simulink library "vmc"  (R2021b)
settings: Solver=VariableStepAuto  StartTime=0.0  StopTime=10.0  RelTol=1e-3
undefined symbols (not defined in the file or in its folder): AVMC_ACCDeltaTqIGain_X_kph, AVMC_ACCDeltaTqIGain_Y_mps2, AVMC_ACCDeltaTqPGain_X_kph, AVMC_ACCDeltaTqPGain_Y_kph, AVMC_ACCLongSteadyCtrl_X_kph, AVMC_AggressJerkPCT4AT_X_kph, AVMC_AggressJerkPCT_X_kph, AVMC_AggressLimitPCT4AT_X_kph, AVMC_AggressLimitPCT_X_kph, AVMC_CCLongSteadyCtrl_X_kph, AVMC_DISCDeltaTqIGain_X_kph, AVMC_DISCDeltaTqIGain_Y_mps2, AVMC_DISCDeltaTqPGain_X_kph, AVMC_DISCDeltaTqPGain_Y_kph, AVMC_DISCTrunAccJerk_X_s, AVMC_DISCTrunAccLimit_X_s, AVMC_ESCRegenOut_X_kph, AVMC_ESCRegenOut_Y_Deg, AVMC_ESCRegenOutEnSpd_X_Deg, AVMC_ISOAccLimit_X_mps, AVMC_ISODecLimit_X_mps, AVMC_ISOJerk_X_mps, AVMC_LatESCRegenOut_X_kph, AVMC_LatESCRegenOut_Y_Deg, AVMC_LongAccDeadZone_X_kph, AVMC_LongAccFiltTsforP2_X_Gps, AVMC_MCPresBaseTq_X_bar, AVMC_MSALongSteadyCtrl_X_kph, AVMC_MSAPedalOvrd2_X_kph, AVMC_MSAPedalOvrd_X_kph, AVMC_MSASpdBand_X_kph, AVMC_MSATqDownEndTq_X_kph, AVMC_MSATqDownTime_X_kph, AVMC_OPDDisSlideRate_X_Deg, AVMC_RDCDetectTime_X_kph, AVMC_RDCDetectTime_Y_pct, AVMC_RDCEnSlideRate_X_Deg, AVMC_RearWhlTqRatio_X_Nm, AVMC_RearWhlTqRatio_Y_gps, AVMC_RearWhlTqSlipGain_X_rat, AVMC_RearWhlTqSlipGain_Y_kph, AVMC_RearWhlTqSTRGGain_X_deg, AVMC_RearWhlTqSTRGGain_Y_kph, AVMC_RWSRrTSA2RWSPos_X_deg, AVMC_RWSSAS2FrtTSA_X_deg, AVMC_RWSVehSPD2RWSCoef_X_kph, AVMC_SoftJerkPCT_X_kph, AVMC_SoftLimitPCT_X_kph, AVMC_StESCYaw_X_kph, AVMC_StESCYaw_Y_Deg, AVMC_StESCYawCom_X_kph, AVMC_StESCYawCom_Y_Gps, AVMC_TMSpdBaseTq_X_rpm, AVMC_VehHoldBDecMap_X_kph, AVMC_VehHoldDecCtrlTime_X_kph, AVMC_VehHoldMCPPass_X_deg, C_TASK_10MS_S, C_TASK_5MS_S, DEG2RAD, ENUM_ACCAVAIL_AVAILABLE ... (+409)
libraries: hcu_lib x74, simulink x68, simulink_extras x3, $bdroot x2
(part 11 of 15)

== system vmc/VMC/VMC/SafetyControl/SafetyControlJudgement ==
  VINP_VehSpeed_kph : Inport
  VVMC_LFWhlSpeedRollAve_kph : Inport  Port=2
  VVMC_RFWhlSpeedRollAve_kph : Inport  Port=3
  VVMC_LRWhlSpeedRollAve_kph : Inport  Port=4
  VVMC_RRWhlSpeedRollAve_kph : Inport  Port=5
  VINP_LFRawWhlSpeedV_flg : Inport  Port=6
  VINP_RFRawWhlSpeedV_flg : Inport  Port=7
  VINP_LRRawWhlSpeedV_flg : Inport  Port=8
  VINP_RRRawWhlSpeedV_flg : Inport  Port=9
  VVMC_LatAccRollAve_Gps : Inport  Port=10
  VINP_LatAccelV_flg : Inport  Port=11
  VVMC_FeatArbitrFinal_enum : Inport  Port=12
  Cast To Single{,1..3} (4 alike) : DataTypeConversion  OutDataTypeStr=boolean
  Constant18 : Constant  Value=C_TASK_10MS_S
  Constant20 : Constant  Value=KVMC_SafetyCtrlAllowTime_s
  Constant21 : Constant  Value=TRUE
  Constant22 : Constant  Value=FALSE
  FrontRearSlipRatio : Subsystem
  LateralAccelerationControl : Subsystem
  NOT : Logic  Operator=NOT  AllPortsSameDT=off  OutDataTypeStr=boolean
  RearWheelSlipRatio : Subsystem
  Relational Operator16 : RelationalOperator  OutDataTypeStr=boolean  RndMeth=Simplest
  SafetyControlJudgement : Subsystem
  SingleWheelSlipRatio : Subsystem
  Timer : hcu_lib/Basic_Blocks/Timer
  u2 > 0 (1) : Switch  Criteria=u2 > Threshold
  VVMC_SafetyCtrl_flg : Outport
  VVMC_FrontRearSlipRatioCtrl_flg : Outport  Port=2
  VVMC_RearWhlSlipRatioCtrl_flg : Outport  Port=3
  VVMC_SingleWhlSlipRatioCtrl_flg : Outport  Port=4
  VVMC_LatAccCtrl_flg : Outport  Port=5
  wires:
  [VVMC_FeatArbitrFinal_enum] -> SafetyControlJudgement/5(VVMC_FeatArbitrFinal_enum)
  VVMC_FeatArbitrFinal_enum/1 -> [VVMC_FeatArbitrFinal_enum]
  Constant18/1 -> Timer/3
  Constant22/1 -> u2 > 0 (1)/3
  Relational Operator16/1 -> u2 > 0 (1)/2
  Timer/1 -> Relational Operator16/1
  Constant20/1 -> Relational Operator16/2, Timer/4
  Constant21/1 -> u2 > 0 (1)/1
  SafetyControlJudgement/1("VVMC_SafetyCtrl_flg ") -> NOT/1, Timer/1
  NOT/1 -> Timer/2
  u2 > 0 (1)/1 -> [VVMC_SafetyCtrl_flg]
  [VVMC_LatAccCtrl_flg] -> VVMC_LatAccCtrl_flg/1
  [VVMC_SingleWhlSlipRatioCtrl_flg] -> VVMC_SingleWhlSlipRatioCtrl_flg/1
  [VVMC_RearWhlSlipRatioCtrl_flg] -> VVMC_RearWhlSlipRatioCtrl_flg/1
  [VVMC_FrontRearSlipRatioCtrl_flg] -> VVMC_FrontRearSlipRatioCtrl_flg/1
  [VVMC_LatAccCtrl_flg] -> SafetyControlJudgement/4(VVMC_LatAccCtrl_flg)
  Cast To Single3/1 -> [VVMC_LatAccCtrl_flg]  "VVMC_LatAccCtrl_flg"
  LateralAccelerationControl/1(VVMC_LatAccCtrl_flg) -> Cast To Single3/1
  [VINP_LatAccelV_flg] -> LateralAccelerationControl/2(VINP_LatAccelV_flg)
  [VVMC_LatAccRollAve_Gps] -> LateralAccelerationControl/1(VVMC_LatAccRollAve_Gps)
  VVMC_LatAccRollAve_Gps/1 -> [VVMC_LatAccRollAve_Gps]
  VINP_LatAccelV_flg/1 -> [VINP_LatAccelV_flg]
  Cast To Single2/1 -> [VVMC_SingleWhlSlipRatioCtrl_flg]  "VVMC_SingleWhlSlipRatioCtrl_flg"
  Cast To Single1/1 -> [VVMC_RearWhlSlipRatioCtrl_flg]  "VVMC_RearWhlSlipRatioCtrl_flg"
  Cast To Single/1 -> [VVMC_FrontRearSlipRatioCtrl_flg]  "VVMC_FrontRearSlipRatioCtrl_flg"
  [VVMC_SafetyCtrl_flg] -> VVMC_SafetyCtrl_flg/1
  [VVMC_SingleWhlSlipRatioCtrl_flg] -> SafetyControlJudgement/3(VVMC_SingleWhlSlipRatioCtrl_flg)
  [VVMC_RearWhlSlipRatioCtrl_flg] -> SafetyControlJudgement/2(VVMC_RearWhlSlipRatioCtrl_flg)
  [VVMC_FrontRearSlipRatioCtrl_flg] -> SafetyControlJudgement/1(VVMC_FrontRearSlipRatioCtrl_flg)
  [VINP_VehSpeed_kph] -> SingleWheelSlipRatio/1(VINP_VehSpeed_kph)
  [VVMC_LFWhlSpeedRollAve_kph] -> SingleWheelSlipRatio/2(VVMC_LFWhlSpeedRollAve_kph)
  [VVMC_RFWhlSpeedRollAve_kph] -> SingleWheelSlipRatio/3(VVMC_RFWhlSpeedRollAve_kph)
  [VVMC_LRWhlSpeedRollAve_kph] -> SingleWheelSlipRatio/4(VVMC_LRWhlSpeedRollAve_kph)
  [VVMC_RRWhlSpeedRollAve_kph] -> SingleWheelSlipRatio/5(VVMC_RRWhlSpeedRollAve_kph)
  [VINP_LFRawWhlSpeedV_flg] -> SingleWheelSlipRatio/6(VINP_LFRawWhlSpeedV_flg)
  [VINP_RFRawWhlSpeedV_flg] -> SingleWheelSlipRatio/7(VINP_RFRawWhlSpeedV_flg)
  [VINP_LRRawWhlSpeedV_flg] -> SingleWheelSlipRatio/8(VINP_LRRawWhlSpeedV_flg)
  [VINP_RRRawWhlSpeedV_flg] -> SingleWheelSlipRatio/9(VINP_RRRawWhlSpeedV_flg)
  SingleWheelSlipRatio/1(VVMC_SingleWhlSlipRatioCtrl_flg) -> Cast To Single2/1
  [VVMC_LRWhlSpeedRollAve_kph] -> RearWheelSlipRatio/1(VVMC_LRWhlSpeedRollAve_kph)
  [VVMC_RRWhlSpeedRollAve_kph] -> RearWheelSlipRatio/2(VVMC_RRWhlSpeedRollAve_kph)
  [VINP_LRRawWhlSpeedV_flg] -> RearWheelSlipRatio/3(VINP_LRRawWhlSpeedV_flg)
  [VINP_RRRawWhlSpeedV_flg] -> RearWheelSlipRatio/4(VINP_RRRawWhlSpeedV_flg)
  RearWheelSlipRatio/1("VVMC_RearWhlSlipRatioCtrl_flg ") -> Cast To Single1/1
  FrontRearSlipRatio/1("VVMC_FrontRearSlipRatioCtrl_flg ") -> Cast To Single/1
  [VINP_RRRawWhlSpeedV_flg] -> FrontRearSlipRatio/8(VINP_RRRawWhlSpeedV_flg)
  [VINP_LRRawWhlSpeedV_flg] -> FrontRearSlipRatio/7(VINP_LRRawWhlSpeedV_flg)
  [VINP_RFRawWhlSpeedV_flg] -> FrontRearSlipRatio/6(VINP_RFRawWhlSpeedV_flg)
  [VINP_LFRawWhlSpeedV_flg] -> FrontRearSlipRatio/5(VINP_LFRawWhlSpeedV_flg)
  [VVMC_RRWhlSpeedRollAve_kph] -> FrontRearSlipRatio/4(VVMC_RRWhlSpeedRollAve_kph)
  [VVMC_LRWhlSpeedRollAve_kph] -> FrontRearSlipRatio/3(VVMC_LRWhlSpeedRollAve_kph)
  [VVMC_RFWhlSpeedRollAve_kph] -> FrontRearSlipRatio/2(VVMC_RFWhlSpeedRollAve_kph)
  [VVMC_LFWhlSpeedRollAve_kph] -> FrontRearSlipRatio/1(VVMC_LFWhlSpeedRollAve_kph)
  VINP_RRRawWhlSpeedV_flg/1 -> [VINP_RRRawWhlSpeedV_flg]
  VINP_LRRawWhlSpeedV_flg/1 -> [VINP_LRRawWhlSpeedV_flg]
  VINP_RFRawWhlSpeedV_flg/1 -> [VINP_RFRawWhlSpeedV_flg]
  VINP_LFRawWhlSpeedV_flg/1 -> [VINP_LFRawWhlSpeedV_flg]
  VVMC_LFWhlSpeedRollAve_kph/1 -> [VVMC_LFWhlSpeedRollAve_kph]
  VVMC_RFWhlSpeedRollAve_kph/1 -> [VVMC_RFWhlSpeedRollAve_kph]
  VVMC_LRWhlSpeedRollAve_kph/1 -> [VVMC_LRWhlSpeedRollAve_kph]
  VVMC_RRWhlSpeedRollAve_kph/1 -> [VVMC_RRWhlSpeedRollAve_kph]
  VINP_VehSpeed_kph/1 -> [VINP_VehSpeed_kph]

== system vmc/VMC/VMC/SafetyControl/VehSpdRollingAverage ==
  VINP_VehSpeed_kph : Inport
  Constant3 : Constant  Value=ONE_INT
  Constant4 : Constant  Value=KVMC_VehSpdRollAveLevel_enum
  Constant5 : Constant  Value=ZERO_FLOAT
  RollingAverage : Stateflow chart  TreatAsAtomicUnit=on
  VVMC_VehSpdRollAve_kph : Outport
  wires:
  [VVMC_VehSpdRollAve_kph] -> VVMC_VehSpdRollAve_kph/1
  VINP_VehSpeed_kph/1 -> [VINP_VehSpeed_kph]  "VINP_VehSpeed_kph"
  RollingAverage/1(VVMC_VehSpdRollAve_kph) -> [VVMC_VehSpdRollAve_kph]  "VVMC_VehSpdRollAve_kph"
  [VINP_VehSpeed_kph] -> RollingAverage/4(VINP_VehSpeed_kph)
  Constant3/1 -> RollingAverage/3(ONE_INT)
  Constant5/1 -> RollingAverage/2(ZERO_FLOAT)
  Constant4/1 -> RollingAverage/1(KVMC_VehSpdRollAveLevel_enum)

== system vmc/VMC/VMC/SafetyControl/WheelSpeedRollingAverage ==
  VINP_LFRawWhlSpeed_kph : Inport
  VINP_RFRawWhlSpeed_kph : Inport  Port=2
  VINP_LRRawWhlSpeed_kph : Inport  Port=3
  VINP_RRRawWhlSpeed_kph : Inport  Port=4
  Constant{3,7,12,16} (4 alike) : Constant  Value=ONE_INT
  Constant{4,8,13,17} (4 alike) : Constant  Value=KVMC_WhlSpdRollAveLevel_enum
  Constant{5,9,14,18} (4 alike) : Constant  Value=ZERO_FLOAT
  RollingAverage : Stateflow chart  TreatAsAtomicUnit=on
  RollingAverage1 : Stateflow chart  TreatAsAtomicUnit=on
  RollingAverage2 : Stateflow chart  TreatAsAtomicUnit=on
  RollingAverage3 : Stateflow chart  TreatAsAtomicUnit=on
  VVMC_LFWhlSpeedRollAve_kph : Outport
  VVMC_RFWhlSpeedRollAve_kph : Outport  Port=2
  VVMC_LRWhlSpeedRollAve_kph : Outport  Port=3
  VVMC_RRWhlSpeedRollAve_kph : Outport  Port=4
  wires:
  [VVMC_RRWhlSpeedRollAve_kph] -> VVMC_RRWhlSpeedRollAve_kph/1
  [VVMC_LRWhlSpeedRollAve_kph] -> VVMC_LRWhlSpeedRollAve_kph/1
  [VVMC_RFWhlSpeedRollAve_kph] -> VVMC_RFWhlSpeedRollAve_kph/1
  [VVMC_LFWhlSpeedRollAve_kph] -> VVMC_LFWhlSpeedRollAve_kph/1
  VINP_RFRawWhlSpeed_kph/1 -> [VINP_RFRawWhlSpeed_kph]
  VINP_LFRawWhlSpeed_kph/1 -> [VINP_LFRawWhlSpeed_kph]
  VINP_RRRawWhlSpeed_kph/1 -> [VINP_RRRawWhlSpeed_kph]
  VINP_LRRawWhlSpeed_kph/1 -> [VINP_LRRawWhlSpeed_kph]
  Constant4/1 -> RollingAverage/1(KVMC_WhlSpdRollAveLevel_enum)
  Constant5/1 -> RollingAverage/2(ZERO_FLOAT)
  Constant3/1 -> RollingAverage/3(ONE_INT)
  [VINP_LFRawWhlSpeed_kph] -> RollingAverage/4(VINP_LFRawWhlSpeed_kph)
  RollingAverage/1(VVMC_LFWhlSpeedRollAve_kph) -> [VVMC_LFWhlSpeedRollAve_kph]
  [VINP_RFRawWhlSpeed_kph] -> RollingAverage1/4(VINP_RFRawWhlSpeed_kph)
  Constant7/1 -> RollingAverage1/3(ONE_INT)
  Constant9/1 -> RollingAverage1/2(ZERO_FLOAT)
  Constant8/1 -> RollingAverage1/1(KVMC_WhlSpdRollAveLevel_enum)
  Constant17/1 -> RollingAverage3/1(KVMC_WhlSpdRollAveLevel_enum)
  Constant18/1 -> RollingAverage3/2(ZERO_FLOAT)
  Constant16/1 -> RollingAverage3/3(ONE_INT)
  [VINP_RRRawWhlSpeed_kph] -> RollingAverage3/4(VINP_RRRawWhlSpeed_kph)
  RollingAverage2/1(VVMC_LRWhlSpeedRollAve_kph) -> [VVMC_LRWhlSpeedRollAve_kph]
  [VINP_LRRawWhlSpeed_kph] -> RollingAverage2/4(VINP_LRRawWhlSpeed_kph)
  Constant12/1 -> RollingAverage2/3(ONE_INT)
  Constant14/1 -> RollingAverage2/2(ZERO_FLOAT)
  Constant13/1 -> RollingAverage2/1(KVMC_WhlSpdRollAveLevel_enum)
  RollingAverage1/1(VVMC_RFWhlSpeedRollAve_kph) -> [VVMC_RFWhlSpeedRollAve_kph]
  RollingAverage3/1(VVMC_RRWhlSpeedRollAve_kph) -> [VVMC_RRWhlSpeedRollAve_kph]

== system vmc/VMC/VMC/Slide Rate  Calculation/4Wheel Calculation ==
  VINP_LFRawWhlSpeed_kph : Inport
  VINP_RFRawWhlSpeed_kph : Inport  Port=2
  VINP_LRRawWhlSpeed_kph : Inport  Port=3
  VINP_RRRawWhlSpeed_kph : Inport  Port=4
  VVMC_LongAcc_Gps : Inport  Port=5
  task_time_s : Inport  Port=6
  VINP_VehSpeed_kph : Inport  Port=7
  VTQD_AfterAvailableTqDemFr_Nm : Inport  Port=8
  VTQD_AfterAvailableTqDemRr_Nm : Inport  Port=9
  VTQD_GearActualPosn_enum : Inport  Port=10
  VINP_LongAccel_Gps : Inport  Port=11
  Constant3 : Constant  Value=KVMC_4WheelLongAccSW_flg
  Determination : Subsystem
  LF Wheel : Subsystem
  LR Wheel : Subsystem
  RF Wheel : Subsystem
  RR Wheel : Subsystem
  Switch : Switch  Criteria=u2 > Threshold
  VVMC_LF4WhlSpdSlideRate_pct : Outport
  VVMC_RF4WhlSpdSlideRate_pct : Outport  Port=2
  VVMC_LR4WhlSpdSlideRate_pct : Outport  Port=3
  VVMC_RR4WhlSpdSlideRate_pct : Outport  Port=4
  VVMC_PredictVehSpd_kph : Outport  Port=5
  VVMC_4WhlSpdSlideRate_pct : Outport  Port=6
  VVMC_AllWhlSkid_flg : Outport  Port=7
  wires:
  [VVMC_4WhlSpdSlideRate_pct] -> VVMC_4WhlSpdSlideRate_pct/1
  [VVMC_PredictVehSpd_kph] -> VVMC_PredictVehSpd_kph/1
  VINP_VehSpeed_kph/1 -> [VINP_VehSpeed_kph]
  task_time_s/1 -> [task_time_s]
  [VVMC_LR4WhlSpdSlideRate_pct] -> VVMC_LR4WhlSpdSlideRate_pct/1
  [VVMC_RR4WhlSpdSlideRate_pct] -> VVMC_RR4WhlSpdSlideRate_pct/1
  [VVMC_RF4WhlSpdSlideRate_pct] -> VVMC_RF4WhlSpdSlideRate_pct/1
  [VVMC_LF4WhlSpdSlideRate_pct] -> VVMC_LF4WhlSpdSlideRate_pct/1
  VINP_LRRawWhlSpeed_kph/1 -> [VINP_LRRawWhlSpeed_kph]
  VINP_LFRawWhlSpeed_kph/1 -> [VINP_LFRawWhlSpeed_kph]
  VINP_RFRawWhlSpeed_kph/1 -> [VINP_RFRawWhlSpeed_kph]
  VINP_RRRawWhlSpeed_kph/1 -> [VINP_RRRawWhlSpeed_kph]
  [VVMC_AllWhlSkid_flg] -> VVMC_AllWhlSkid_flg/1
  VTQD_AfterAvailableTqDemFr_Nm/1 -> [VTQD_AfterAvailableTqDemFr_Nm]
  VTQD_AfterAvailableTqDemRr_Nm/1 -> [VTQD_AfterAvailableTqDemRr_Nm]
  VTQD_GearActualPosn_enum/1 -> [VTQD_GearActualPosn_enum]
  [VVMC_LRPreVehSpd_kph] -> Determination/17(VVMC_LRPreVehSpd_kph)
  [VVMC_4WheelLongAcc_Gps] -> LF Wheel/1(VVMC_4WheelLongAcc_Gps)
  [VINP_RRRawWhlSpeed_kph] -> RR Wheel/3(VINP_RRRawWhlSpeed_kph)
  [VINP_LRRawWhlSpeed_kph] -> LR Wheel/3(VINP_LRRawWhlSpeed_kph)
  [VINP_RFRawWhlSpeed_kph] -> RF Wheel/3(VINP_RFRawWhlSpeed_kph)
  [VTQD_GearActualPosn_enum] -> RF Wheel/4(VTQD_GearActualPosn_enum)
  LF Wheel/1(VVMC_LFPreVehSpd_kph) -> [VVMC_LFPreVehSpd_kph]
  RR Wheel/1(VVMC_RRPreVehSpd_kph) -> [VVMC_RRPreVehSpd_kph]
  [VTQD_GearActualPosn_enum] -> LR Wheel/4(VTQD_GearActualPosn_enum)
  [VVMC_LF4WhlSpdSlideRate_pct] -> Determination/9(VVMC_LF4WhlSpdSlideRate_pct)
  [VVMC_RRWhlSkid_flg] -> Determination/8(VVMC_RRWhlSkid_flg)
  [VINP_LFRawWhlSpeed_kph] -> LF Wheel/3(VINP_LFRawWhlSpeed_kph)
  [task_time_s] -> RR Wheel/2(task_time_s)
  [task_time_s] -> RF Wheel/2(task_time_s)
  [VVMC_RR4WhlSpdSlideRate_pct] -> Determination/12(VVMC_RR4WhlSpdSlideRate_pct)
  RR Wheel/3(VVMC_RR4WhlSpdSlideRate_pct) -> [VVMC_RR4WhlSpdSlideRate_pct]
  [VTQD_AfterAvailableTqDemFr_Nm] -> Determination/13(VTQD_AfterAvailableTqDemFr_Nm)
  [VVMC_LR4WhlSpdSlideRate_pct] -> Determination/11(VVMC_LR4WhlSpdSlideRate_pct)
  [VTQD_GearActualPosn_enum] -> Determination/4(VTQD_GearActualPosn_enum)
  [task_time_s] -> Determination/2(task_time_s)
  [VVMC_LFWhlSkid_flg] -> Determination/5(VVMC_LFWhlSkid_flg)
  [VINP_VehSpeed_kph] -> Determination/3(VINP_VehSpeed_kph)
  [VVMC_RRPreVehSpd_kph] -> Determination/18(VVMC_RRPreVehSpd_kph)
  Determination/2(VVMC_AllWhlSkid_flg) -> [VVMC_AllWhlSkid_flg]
  Determination/1(VVMC_PredictVehSpd_kph) -> [VVMC_PredictVehSpd_kph]
  Determination/3(VVMC_4WhlSpdSlideRate_pct) -> [VVMC_4WhlSpdSlideRate_pct]
  [VVMC_RFWhlSkid_flg] -> Determination/6(VVMC_RFWhlSkid_flg)
  LR Wheel/3(VVMC_LR4WhlSpdSlideRate_pct) -> [VVMC_LR4WhlSpdSlideRate_pct]
  LR Wheel/2(VVMC_LRWhlSkid_flg) -> [VVMC_LRWhlSkid_flg]
  [VVMC_LRWhlSkid_flg] -> Determination/7(VVMC_LRWhlSkid_flg)
  RF Wheel/1(VVMC_RFPreVehSpd_kph) -> [VVMC_RFPreVehSpd_kph]
  [task_time_s] -> LR Wheel/2(task_time_s)
  [VVMC_RFPreVehSpd_kph] -> Determination/16(VVMC_RFPreVehSpd_kph)
  LR Wheel/1(VVMC_LRPreVehSpd_kph) -> [VVMC_LRPreVehSpd_kph]
  [VVMC_4WheelLongAcc_Gps] -> RF Wheel/1(VVMC_4WheelLongAcc_Gps)
  RR Wheel/2(VVMC_RRWhlSkid_flg) -> [VVMC_RRWhlSkid_flg]
  [VVMC_LFPreVehSpd_kph] -> Determination/15(VVMC_LFPreVehSpd_kph)
  [VVMC_RF4WhlSpdSlideRate_pct] -> Determination/10(VVMC_RF4WhlSpdSlideRate_pct)
  [VTQD_AfterAvailableTqDemRr_Nm] -> Determination/14(VTQD_AfterAvailableTqDemRr_Nm)
  LF Wheel/2(VVMC_LFWhlSkid_flg) -> [VVMC_LFWhlSkid_flg]
  RF Wheel/2(VVMC_RFWhlSkid_flg) -> [VVMC_RFWhlSkid_flg]
  [VVMC_4WheelLongAcc_Gps] -> Determination/1(VVMC_4WheelLongAcc_Gps)
  [VVMC_4WheelLongAcc_Gps] -> RR Wheel/1(VVMC_4WheelLongAcc_Gps)
  [VTQD_GearActualPosn_enum] -> RR Wheel/4(VTQD_GearActualPosn_enum)
  [VVMC_4WheelLongAcc_Gps] -> LR Wheel/1(VVMC_4WheelLongAcc_Gps)
  RF Wheel/3(VVMC_RF4WhlSpdSlideRate_pct) -> [VVMC_RF4WhlSpdSlideRate_pct]
  LF Wheel/3(VVMC_LF4WhlSpdSlideRate_pct) -> [VVMC_LF4WhlSpdSlideRate_pct]
  [task_time_s] -> LF Wheel/2(task_time_s)
  [VTQD_GearActualPosn_enum] -> LF Wheel/4(VTQD_GearActualPosn_enum)
  Constant3/1 -> Switch/2
  Switch/1 -> [VVMC_4WheelLongAcc_Gps]  "VVMC_4WheelLongAcc_Gps"
  VINP_LongAccel_Gps/1 -> [VINP_LongAccel_Gps]
  VVMC_LongAcc_Gps/1 -> [VVMC_LongAcc_Gps]
  [VVMC_LongAcc_Gps] -> Switch/3
  [VINP_LongAccel_Gps] -> Switch/1

== system vmc/VMC/VMC/Slide Rate  Calculation/Alternative Wheel Slide Calculation ==
  VINP_LFRawWhlSpeed_kph : Inport
  VINP_RFRawWhlSpeed_kph : Inport  Port=2
  VINP_LRRawWhlSpeed_kph : Inport  Port=3
  VINP_RRRawWhlSpeed_kph : Inport  Port=4
  Abs : Abs
  Abs1 : Abs
  Add : Sum  Inputs=+-
  Add1 : Sum  Inputs=+-
  Constant{,3,5,8} (4 alike) : Constant  Value=KVMC_RawWhlSpeedDeadZone_kph
  Constant1 : Constant  Value=ONE_FLOAT
  Constant2 : Constant  Value=ONE_PERCENT
  Constant4 : Constant  Value=ZERO_FLOAT
  Constant6 : Constant  Value=ONE_FLOAT
  Constant7 : Constant  Value=ONE_PERCENT
  Constant9 : Constant  Value=ZERO_FLOAT
  Divide : Product  Inputs=*//
  Divide1 : Product  Inputs=*//
  Relational Operator{,1..3} (4 alike) : RelationalOperator  Operator=<=  OutDataTypeStr=boolean  RndMeth=Simplest
  Relational Operator4 : RelationalOperator  OutDataTypeStr=boolean  RndMeth=Simplest
  Switch{,1..4} (5 alike) : Switch  Criteria=u2 > Threshold
  VVMC_AltLWhlSlideRate_pct : Outport
  VVMC_AltRWhlSlideRate_pct : Outport  Port=2
  VVMC_AltWhlSlideRate_pct : Outport  Port=3
  wires:
  VINP_RRRawWhlSpeed_kph/1 -> [VINP_RRRawWhlSpeed_kph]
  Relational Operator1/1 -> Switch1/2
  Abs/1 -> Relational Operator4/1
  Divide/1 -> Switch1/3  "VVMC_CalAltLWhlSlideRate_pct"
  Constant1/1 -> Switch/1
  [VINP_LFRawWhlSpeed_kph] -> Add/2
  Switch1/1 -> [VVMC_AltLWhlSlideRate_pct]  "VVMC_AltLWhlSlideRate_pct"
  Constant6/1 -> Switch2/1
  Relational Operator3/1 -> Switch3/2
  Relational Operator4/1 -> Switch4/2
  [VVMC_AltLWhlSlideRate_pct] -> Abs/1
  [VVMC_AltLWhlSlideRate_pct] -> VVMC_AltLWhlSlideRate_pct/1
  VINP_LFRawWhlSpeed_kph/1 -> [VINP_LFRawWhlSpeed_kph]
  VINP_LRRawWhlSpeed_kph/1 -> [VINP_LRRawWhlSpeed_kph]
  VINP_RFRawWhlSpeed_kph/1 -> [VINP_RFRawWhlSpeed_kph]
  [VVMC_AltRWhlSlideRate_pct] -> Switch4/3
  Switch3/1 -> [VVMC_AltRWhlSlideRate_pct]  "VVMC_AltRWhlSlideRate_pct"
  Constant4/1 -> Switch1/1
  Constant3/1 -> Relational Operator1/2
  [VVMC_AltRWhlSlideRate_pct] -> Abs1/1
  [VVMC_AltLWhlSlideRate_pct] -> Switch4/1
  Switch4/1 -> [VVMC_AltWhlSlideRate_pct]  "VVMC_AltWhlSlideRate_pct"
  Constant2/1 -> Divide/2
  Constant7/1 -> Divide1/2
  Switch/1 -> Divide/3
  Constant9/1 -> Switch3/1
  [VINP_LFRawWhlSpeed_kph] -> Switch/3
  Relational Operator/1 -> Switch/2
  [VVMC_AltWhlSlideRate_pct] -> VVMC_AltWhlSlideRate_pct/1
  [VINP_RFRawWhlSpeed_kph] -> Add1/2
  Add/1 -> Divide/1
  Constant/1 -> Relational Operator/2
  [VINP_LFRawWhlSpeed_kph] -> Relational Operator1/1
  Abs1/1 -> Relational Operator4/2
  [VINP_RRRawWhlSpeed_kph] -> Add1/1
  [VINP_RFRawWhlSpeed_kph] -> Relational Operator3/1
  [VINP_RFRawWhlSpeed_kph] -> Switch2/3
  Add1/1 -> Divide1/1
  [VINP_LFRawWhlSpeed_kph] -> Relational Operator/1
  [VINP_LRRawWhlSpeed_kph] -> Add/1
  [VINP_RFRawWhlSpeed_kph] -> Relational Operator2/1
  Constant8/1 -> Relational Operator3/2
  Constant5/1 -> Relational Operator2/2
  Divide1/1 -> Switch3/3  "VVMC_CalAltRWhlSlideRate_pct"
  Switch2/1 -> Divide1/3
  Relational Operator2/1 -> Switch2/2
  [VVMC_AltRWhlSlideRate_pct] -> VVMC_AltRWhlSlideRate_pct/1

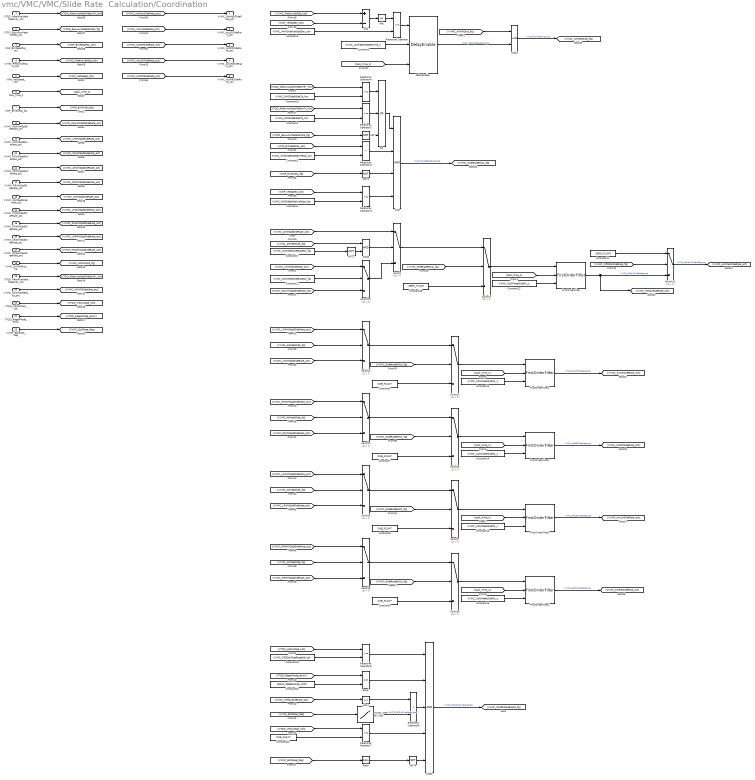
== system vmc/VMC/VMC/Slide Rate  Calculation/Coordination ==
  VTQD_AfterAvailableTqDemFr_Nm : Inport
  VTQD_EquivAccPedalSWSta_flg : Inport  Port=2
  VINP_BrkPedalPos_pct : Inport  Port=3
  VVMC_PredictVehSpd_kph : Inport  Port=4
  VINP_VehSpeed_kph : Inport  Port=5
  task_time_s : Inport  Port=6
  VINP_BrkSwSta_flg : Inport  Port=7
  VVMC_RawWhlSpdSlideRate_pct : Inport  Port=8
  VVMC_LFWhlSpdSlideRate_pct : Inport  Port=9
  VVMC_RFWhlSpdSlideRate_pct : Inport  Port=10
  VVMC_LRWhlSpdSlideRate_pct : Inport  Port=11
  VVMC_RRWhlSpdSlideRate_pct : Inport  Port=12
  VVMC_4WhlSpdSlideRate_pct : Inport  Port=13
  VVMC_LF4WhlSpdSlideRate_pct : Inport  Port=14
  VVMC_RF4WhlSpdSlideRate_pct : Inport  Port=15
  VVMC_LR4WhlSpdSlideRate_pct : Inport  Port=16
  VVMC_RR4WhlSpdSlideRate_pct : Inport  Port=17
  VVMC_AllWhlSkid_flg : Inport  Port=18
  VTQD_AfterAvailableTqDemRr_Nm : Inport  Port=19
  VVMC_AltWhlSlideRate_pct : Inport  Port=20
  VTQD_VehActSpd_kph : Inport  Port=21
  VTQD_RegenMode_enum : Inport  Port=22
  VVMC_EstSlope_Deg : Inport  Port=23
  AND : Logic  Inputs=4  AllPortsSameDT=off  OutDataTypeStr=boolean
  AND1 : Logic  AllPortsSameDT=off  OutDataTypeStr=boolean
  AND2 : Logic  AllPortsSameDT=off  OutDataTypeStr=boolean
  AND3 : Logic  Inputs=5  AllPortsSameDT=off  OutDataTypeStr=boolean
  Abs : Abs
  Abs1 : Abs
  Add : Sum  Inputs=+-
  Constant1 : Constant  Value=KVMC_WhlSlideEnDetTq_Nm
  Constant10 : Constant  Value=KVMC_WhlSlideEnDetTq_Nm
  Constant11 : Constant  Value=KVMC_AltWheelSlideRateSW_flg
  Constant{12..16} (5 alike) : Constant  Value=KVMC_CalWhleelSlideTs_c
  Constant17 : Constant  Value=KVMC_AltWheelSlideRateSW_flg
  Constant18 : Constant  Value=ZERO_FLOAT
  Constant19 : Constant  Value=KVMC_OPDDisSlideRateSpd_kph
  Constant2 : Constant  Value=KVMC_WhlSlideEnDetBrkPedal_pct
  Constant20 : Constant  Value=ENUM_REGENLEVEL_OPD
  Constant21 : Constant  Value=ZERO_FLOAT
  Constant{6..9,22} (5 alike) : Constant  Value=ONE_FLOAT
  Constant3 : Constant  Value=KVMC_4WhlSlideVehSpdDev_kph
  Constant4 : Constant  Value=KVMC_WhlSlideEnDetVehSpd_kph
  Constant5 : Constant  Value=KVMC_4WhleelSlideDetTime_s
  DelayEnable : hcu_lib/Basic_Blocks/DelayEnable
  Equal : RelationalOperator  Operator===  OutDataTypeStr=boolean  RndMeth=Simplest
  FirstOrderFilter{,1..4} (5 alike) : hcu_lib/Basic_Blocks/FirstOrderFilter
  MVMC_OPDDisSlideRate_Y_pct : Lookup_n-D  NumberOfTableDimensions=1  BreakpointsForDimension1=AVMC_OPDDisSlideRate_X_Deg  Table=MVMC_OPDDisSlideRate_Y_pct  InternalRulePriority=Speed  RndMeth=Simplest  InputSameDT=on
  NOT{,1..3} (4 alike) : Logic  Operator=NOT  AllPortsSameDT=off  OutDataTypeStr=boolean
  OR : Logic  Operator=OR  Inputs=3  AllPortsSameDT=off  OutDataTypeStr=boolean
  Relational Operator{,1,3..4,7} (5 alike) : RelationalOperator  OutDataTypeStr=boolean  RndMeth=Simplest
  Relational Operator2 : RelationalOperator  Operator=<  OutDataTypeStr=boolean  RndMeth=Simplest
  Relational Operator5 : RelationalOperator  Operator=<=  OutDataTypeStr=boolean  RndMeth=Simplest
  Relational Operator6 : RelationalOperator  Operator=<  OutDataTypeStr=boolean  RndMeth=Simplest
  Relay : Relay  OnSwitchValue=KTQD_OPDHoldGradeUp_Deg  OffSwitchValue=KTQD_OPDHoldGradeDown_Deg  OutDataTypeStr=boolean
  Switch{,1..11} (12 alike) : Switch  Criteria=u2 > Threshold
  VVMC_ActMaxSlideRate_pct : Outport
  VVMC_ActLFSlideRate_pct : Outport  Port=2
  VVMC_ActRFSlideRate_pct : Outport  Port=3
  VVMC_ActLRSlideRate_pct : Outport  Port=4
  VVMC_ActRRSlideRate_pct : Outport  Port=5
  wires:
  VVMC_RR4WhlSpdSlideRate_pct/1 -> [VVMC_RR4WhlSpdSlideRate_pct]
  VVMC_LR4WhlSpdSlideRate_pct/1 -> [VVMC_LR4WhlSpdSlideRate_pct]
  VVMC_RF4WhlSpdSlideRate_pct/1 -> [VVMC_RF4WhlSpdSlideRate_pct]
  VVMC_LF4WhlSpdSlideRate_pct/1 -> [VVMC_LF4WhlSpdSlideRate_pct]
  VVMC_4WhlSpdSlideRate_pct/1 -> [VVMC_4WhlSpdSlideRate_pct]
  VVMC_LRWhlSpdSlideRate_pct/1 -> [VVMC_LRWhlSpdSlideRate_pct]
  VVMC_RRWhlSpdSlideRate_pct/1 -> [VVMC_RRWhlSpdSlideRate_pct]
  VVMC_LFWhlSpdSlideRate_pct/1 -> [VVMC_LFWhlSpdSlideRate_pct]
  VVMC_RFWhlSpdSlideRate_pct/1 -> [VVMC_RFWhlSpdSlideRate_pct]
  VVMC_RawWhlSpdSlideRate_pct/1 -> [VVMC_RawWhlSpdSlideRate_pct]
  task_time_s/1 -> [task_time_s]
  VINP_BrkSwSta_flg/1 -> [VINP_BrkSwSta_flg]
  VINP_VehSpeed_kph/1 -> [VINP_VehSpeed_kph]
  VINP_BrkPedalPos_pct/1 -> [VINP_BrkPedalPos_pct]
  VTQD_EquivAccPedalSWSta_flg/1 -> [VTQD_EquivAccPedalSWSta_flg]
  VTQD_AfterAvailableTqDemFr_Nm/1 -> [VTQD_AfterAvailableTqDemFr_Nm]
  VVMC_PredictVehSpd_kph/1 -> [VVMC_PredictVehSpd_kph]
  [VVMC_ActRFSlideRate_pct] -> VVMC_ActRFSlideRate_pct/1
  [VVMC_ActLFSlideRate_pct] -> VVMC_ActLFSlideRate_pct/1
  [VVMC_ActMaxSlideRate_pct] -> VVMC_ActMaxSlideRate_pct/1
  [VVMC_ActLRSlideRate_pct] -> VVMC_ActLRSlideRate_pct/1
  [VVMC_ActRRSlideRate_pct] -> VVMC_ActRRSlideRate_pct/1
  [VINP_VehSpeed_kph] -> Add/2
  OR/1 -> AND/1
  [VVMC_RRWhlSpdSlideRate_pct] -> Switch8/3
  Constant4/1 -> Relational Operator3/2
  [VVMC_4WheelSlide_flg] -> AND2/1
  [VVMC_4WhlSpdSlideRate_pct] -> Switch/1
  [VVMC_SlideRateEnCal_flg] -> Switch9/2
  [VVMC_4WheelSlide_flg] -> Switch6/2
  [VVMC_LR4WhlSpdSlideRate_pct] -> Switch6/1
  [VTQD_EquivAccPedalSWSta_flg] -> NOT/1
  Constant8/1 -> Switch7/3
  [VVMC_LF4WhlSpdSlideRate_pct] -> Switch2/1
  Abs/1 -> Relational Operator/1
  Switch8/1 -> Switch9/1
  [VVMC_LRWhlSpdSlideRate_pct] -> Switch6/3
  [VVMC_SlideRateEnCal_flg] -> Switch5/2
  Switch/1 -> Switch1/1
  Constant7/1 -> Switch5/3
  Switch4/1 -> Switch5/1
  Constant9/1 -> Switch9/3
  Constant5/1 -> DelayEnable/2
  [VINP_BrkPedalPos_pct] -> Relational Operator2/1
  Switch6/1 -> Switch7/1
  NOT1/1 -> AND/3
  [VVMC_RFWhlSpdSlideRate_pct] -> Switch4/3
  [VVMC_SlideRateEnCal_flg] -> Switch3/2
  Constant18/1 -> Switch1/3
  Constant6/1 -> Switch3/3
  Switch2/1 -> Switch3/1
  [VVMC_RF4WhlSpdSlideRate_pct] -> Switch4/1
  [VVMC_4WheelSlide_flg] -> Switch4/2
  Add/1 -> Abs/1
  [VVMC_4WheelSlide_flg] -> Switch2/2
  Relational Operator/1 -> DelayEnable/1
  [VVMC_4WheelSlide_flg] -> Switch8/2
  [VVMC_RR4WhlSpdSlideRate_pct] -> Switch8/1
  Relational Operator3/1 -> AND/4
  [VVMC_LFWhlSpdSlideRate_pct] -> Switch2/3
  Constant1/1 -> Relational Operator1/2
  [VVMC_PredictVehSpd_kph] -> Add/1
  [VINP_BrkSwSta_flg] -> NOT1/1
  [VINP_VehSpeed_kph] -> Relational Operator3/1
  Relational Operator2/1 -> AND/2
  AND/1 -> [VVMC_SlideRateEnCal_flg]  "VVMC_SlideRateEnCal_flg"
  [VVMC_SlideRateEnCal_flg] -> Switch7/2
  Constant3/1 -> Relational Operator/2
  Constant2/1 -> Relational Operator2/2
  [task_time_s] -> DelayEnable/3
  VVMC_AllWhlSkid_flg/1 -> [VVMC_AllWhlSkid_flg]
  DelayEnable/1 -> AND1/2  "VVMC_VehSpdPredSkid_flg"
  AND1/1 -> [VVMC_4WheelSlide_flg]  "VVMC_4WheelSlide_flg"
  [VVMC_AllWhlSkid_flg] -> AND1/1
  Constant10/1 -> Relational Operator4/2
  [VTQD_AfterAvailableTqDemRr_Nm] -> Relational Operator4/1
  NOT/1 -> OR/3
  Relational Operator1/1 -> OR/2
  Relational Operator4/1 -> OR/1
  [VTQD_AfterAvailableTqDemFr_Nm] -> Relational Operator1/1
  VTQD_AfterAvailableTqDemRr_Nm/1 -> [VTQD_AfterAvailableTqDemRr_Nm]
  VVMC_AltWhlSlideRate_pct/1 -> [VVMC_AltWhlSlideRate_pct]
  [VVMC_RawWhlSpdSlideRate_pct] -> Switch10/3
  Switch10/1 -> Switch/3
  [VVMC_AltWhlSlideRate_pct] -> Switch10/1
  Constant11/1 -> Switch10/2
  Switch1/1 -> FirstOrderFilter/1
  FirstOrderFilter1/1 -> [VVMC_ActLFSlideRate_pct]  "VVMC_ActLFSlideRate_pct"
  Switch3/1 -> FirstOrderFilter1/1
  Switch5/1 -> FirstOrderFilter2/1
  FirstOrderFilter2/1 -> [VVMC_ActRFSlideRate_pct]  "VVMC_ActRFSlideRate_pct"
  Switch7/1 -> FirstOrderFilter3/1
  FirstOrderFilter3/1 -> [VVMC_ActLRSlideRate_pct]  "VVMC_ActLRSlideRate_pct"
  Switch9/1 -> FirstOrderFilter4/1
  FirstOrderFilter4/1 -> [VVMC_ActRRSlideRate_pct]  "VVMC_ActRRSlideRate_pct"
  Constant12/1 -> FirstOrderFilter/3
  [task_time_s] -> FirstOrderFilter/2
  [task_time_s] -> FirstOrderFilter1/2
  Constant13/1 -> FirstOrderFilter1/3
  [task_time_s] -> FirstOrderFilter2/2
  Constant14/1 -> FirstOrderFilter2/3
  Constant15/1 -> FirstOrderFilter3/3
  [task_time_s] -> FirstOrderFilter3/2
  Constant16/1 -> FirstOrderFilter4/3
  [task_time_s] -> FirstOrderFilter4/2
  Constant17/1 -> NOT2/1
  NOT2/1 -> AND2/2
  AND2/1 -> Switch/2
  VVMC_EstSlope_Deg/1 -> [VVMC_EstSlope_Deg]
  VTQD_RegenMode_enum/1 -> [VTQD_RegenMode_enum]
  VTQD_VehActSpd_kph/1 -> [VTQD_VehActSpd_kph]
  [VTQD_VehActSpd_kph] -> Relational Operator5/1
  Constant19/1 -> Relational Operator5/2
  [VTQD_RegenMode_enum] -> Equal/1
  Constant20/1 -> Equal/2
  [VVMC_EstSlope_Deg] -> MVMC_OPDDisSlideRate_Y_pct/1
  MVMC_OPDDisSlideRate_Y_pct/1 -> Relational Operator6/2  "VVMC_OPDDisSlideRate_pct"
  Relational Operator5/1 -> AND3/1
  Equal/1 -> AND3/2
  Relational Operator6/1 -> AND3/3
  AND3/1 -> [VVMC_OPDDisSlideRate_flg]  "VVMC_OPDDisSlideRate_flg"
  [VVMC_IntMaxSlideRate_pct] -> Abs1/1
  Abs1/1 -> Relational Operator6/1
  [VVMC_SlideRateEnCal_flg] -> Switch1/2
  FirstOrderFilter/1 -> [VVMC_IntMaxSlideRate_pct], Switch11/3  "VVMC_IntMaxSlideRate_pct"
  Switch11/1 -> [VVMC_ActMaxSlideRate_pct]  "VVMC_ActMaxSlideRate_pct"
  [VVMC_OPDDisSlideRate_flg] -> Switch11/2
  Constant21/1 -> Switch11/1
  Constant22/1 -> Relational Operator7/2
  [VTQD_VehActSpd_kph] -> Relational Operator7/1
  Relational Operator7/1 -> AND3/4
  NOT3/1 -> AND3/5
  Relay/1 -> NOT3/1
  [VVMC_EstSlope_Deg] -> Relay/1

== system vmc/VMC/VMC/Slide Rate  Calculation/Partial Wheel Calculation ==
  VINP_LFRawWhlSpeed_kph : Inport
  VINP_RFRawWhlSpeed_kph : Inport  Port=2
  VINP_LRRawWhlSpeed_kph : Inport  Port=3
  VINP_RRRawWhlSpeed_kph : Inport  Port=4
  VTQD_AfterAvailableTqDemFr_Nm : Inport  Port=5
  VTQD_AfterAvailableTqDemRr_Nm : Inport  Port=6
  Add{,1..4} (5 alike) : Sum  Inputs=+-
  Add5 : Sum
  Constant{,3,5,8,10,13,15,18,20,23} (10 alike) : Constant  Value=KVMC_RawWhlSpeedDeadZone_kph
  Constant{1,6,11,16,21,26} (6 alike) : Constant  Value=ONE_FLOAT
  Constant{2,7,12,17,22} (5 alike) : Constant  Value=ONE_PERCENT
  Constant{4,9,14,19,24..25} (6 alike) : Constant  Value=ZERO_FLOAT
  Constant27 : Constant  Value=MINUSONE_FLOAT
  Divide{,1..4} (5 alike) : Product  Inputs=*//
  Max : MinMax  Function=max  Inputs=4
  Max1 : MinMax  Inputs=4
  Product : Product
  Relational Operator{,1..10} (11 alike) : RelationalOperator  Operator=<=  OutDataTypeStr=boolean  RndMeth=Simplest
  Switch{,1..10} (11 alike) : Switch  Criteria=u2 > Threshold
  VVMC_RawWhlSpdSlideRate_pct : Outport
  VVMC_LFWhlSpdSlideRate_pct : Outport  Port=2
  VVMC_RFWhlSpdSlideRate_pct : Outport  Port=3
  VVMC_LRWhlSpdSlideRate_pct : Outport  Port=4
  VVMC_RRWhlSpdSlideRate_pct : Outport  Port=5
  wires:
  [VVMC_RRWhlSpdSlideRate_pct] -> VVMC_RRWhlSpdSlideRate_pct/1
  [VVMC_LRWhlSpdSlideRate_pct] -> VVMC_LRWhlSpdSlideRate_pct/1
  [VVMC_LFWhlSpdSlideRate_pct] -> VVMC_LFWhlSpdSlideRate_pct/1
  [VVMC_RFWhlSpdSlideRate_pct] -> VVMC_RFWhlSpdSlideRate_pct/1
  [VVMC_RawWhlSpdSlideRate_pct] -> VVMC_RawWhlSpdSlideRate_pct/1
  VINP_RRRawWhlSpeed_kph/1 -> [VINP_RRRawWhlSpeed_kph]
  VINP_LRRawWhlSpeed_kph/1 -> [VINP_LRRawWhlSpeed_kph]
  VINP_RFRawWhlSpeed_kph/1 -> [VINP_RFRawWhlSpeed_kph]
  VINP_LFRawWhlSpeed_kph/1 -> [VINP_LFRawWhlSpeed_kph]
  Constant15/1 -> Relational Operator6/2
  Relational Operator6/1 -> Switch6/2
  Constant16/1 -> Switch6/1
  Constant17/1 -> Divide3/2
  Switch6/1 -> Divide3/3
  Switch7/1 -> [VVMC_LRWhlSpdSlideRate_pct]  "VVMC_LRWhlSpdSlideRate_pct"
  Relational Operator7/1 -> Switch7/2
  [VINP_LRRawWhlSpeed_kph] -> Relational Operator7/1
  Constant18/1 -> Relational Operator7/2
  [VVMC_MinRawWhlSpeed_kph] -> Switch6/3
  [VVMC_MinRawWhlSpeed_kph] -> Relational Operator6/1
  [VINP_LRRawWhlSpeed_kph] -> Add3/1
  Add3/1 -> Divide3/1
  [VVMC_MinRawWhlSpeed_kph] -> Add3/2
  [VINP_RFRawWhlSpeed_kph] -> Max1/2
  [VINP_LRRawWhlSpeed_kph] -> Max1/3
  Max1/1 -> [VVMC_MinRawWhlSpeed_kph]  "VVMC_MinRawWhlSpeed_kph"
  Add/1 -> Divide/1
  Divide1/1 -> Switch3/3  "VVMC_LFCalWhlSpdSlideRate_pct"
  [VINP_LFRawWhlSpeed_kph] -> Relational Operator3/1
  Switch3/1 -> [VVMC_LFWhlSpdSlideRate_pct]  "VVMC_LFWhlSpdSlideRate_pct"
  Constant8/1 -> Relational Operator3/2
  Constant7/1 -> Divide1/2
  Product/1 -> [VVMC_RawWhlSpdSlideRate_pct]  "VVMC_RawWhlSpdSlideRate_pct"
  Constant2/1 -> Divide/2
  Relational Operator3/1 -> Switch3/2
  [VINP_RRRawWhlSpeed_kph] -> Relational Operator9/1
  [VVMC_MinRawWhlSpeed_kph] -> Switch/3
  Add4/1 -> Divide4/1
  Constant24/1 -> Switch9/1
  [VINP_LFRawWhlSpeed_kph] -> Max/1
  [VINP_RRRawWhlSpeed_kph] -> Max/4
  Constant14/1 -> Switch5/1
  Constant9/1 -> Switch3/1
  Constant21/1 -> Switch8/1
  Constant22/1 -> Divide4/2
  Switch4/1 -> Divide2/3
  Constant12/1 -> Divide2/2
  Divide3/1 -> Switch7/3  "VVMC_LRCalWhlSpdSlideRate_pct"
  Constant11/1 -> Switch4/1
  [VINP_RFRawWhlSpeed_kph] -> Add2/1
  [VINP_RFRawWhlSpeed_kph] -> Max/2
  Relational Operator4/1 -> Switch4/2
  Add2/1 -> Divide2/1
  [VVMC_MinRawWhlSpeed_kph] -> Add2/2
  [VVMC_MaxRawWhlSpeed_kph] -> Add/1
  [VINP_LRRawWhlSpeed_kph] -> Max/3
  [VVMC_MinRawWhlSpeed_kph] -> Relational Operator4/1
  Relational Operator1/1 -> Switch1/2
  Switch2/1 -> Divide1/3
  Divide2/1 -> Switch5/3  "VVMC_RFCalWhlSpdSlideRate_pct"
  [VINP_RRRawWhlSpeed_kph] -> Max1/4
  [VVMC_MinRawWhlSpeed_kph] -> Switch4/3
  Constant6/1 -> Switch2/1
  Max/1 -> [VVMC_MaxRawWhlSpeed_kph]  "VVMC_MaxRawWhlSpeed_kph"
  Constant19/1 -> Switch7/1
  [VINP_LFRawWhlSpeed_kph] -> Max1/1
  [VVMC_MinRawWhlSpeed_kph] -> Switch2/3
  [VINP_LFRawWhlSpeed_kph] -> Add1/1
  Constant13/1 -> Relational Operator5/2
  Constant23/1 -> Relational Operator9/2
  Add1/1 -> Divide1/1
  Constant3/1 -> Relational Operator1/2
  [VINP_RRRawWhlSpeed_kph] -> Add4/1
  Relational Operator2/1 -> Switch2/2
  Switch9/1 -> [VVMC_RRWhlSpdSlideRate_pct]  "VVMC_RRWhlSpdSlideRate_pct"
  [VVMC_MinRawWhlSpeed_kph] -> Switch8/3
  [VINP_RFRawWhlSpeed_kph] -> Relational Operator5/1
  [VVMC_MinRawWhlSpeed_kph] -> Relational Operator2/1
  Constant10/1 -> Relational Operator4/2
  Constant/1 -> Relational Operator/2
  Divide4/1 -> Switch9/3  "VVMC_RRCalWhlSpdSlideRate_pct"
  Relational Operator/1 -> Switch/2
  [VVMC_MaxRawWhlSpeed_kph] -> Relational Operator1/1
  [VVMC_MinRawWhlSpeed_kph] -> Add1/2
  [VVMC_MinRawWhlSpeed_kph] -> Add4/2
  Constant1/1 -> Switch/1
  Constant20/1 -> Relational Operator8/2
  Relational Operator9/1 -> Switch9/2
  Switch/1 -> Divide/3
  Switch8/1 -> Divide4/3
  Constant4/1 -> Switch1/1
  Switch5/1 -> [VVMC_RFWhlSpdSlideRate_pct]  "VVMC_RFWhlSpdSlideRate_pct"
  [VVMC_MinRawWhlSpeed_kph] -> Add/2
  Relational Operator5/1 -> Switch5/2
  Relational Operator8/1 -> Switch8/2
  Divide/1 -> Switch1/3  "VVMC_RawCalWhlSpdSlideRate_pct"
  Constant5/1 -> Relational Operator2/2
  [VVMC_MinRawWhlSpeed_kph] -> Relational Operator/1
  [VVMC_MinRawWhlSpeed_kph] -> Relational Operator8/1
  VTQD_AfterAvailableTqDemFr_Nm/1 -> [VTQD_AfterAvailableTqDemFr_Nm]
  VTQD_AfterAvailableTqDemRr_Nm/1 -> [VTQD_AfterAvailableTqDemRr_Nm]
  Relational Operator10/1 -> Switch10/2
  Constant27/1 -> Switch10/1
  [VTQD_AfterAvailableTqDemRr_Nm] -> Add5/2
  [VTQD_AfterAvailableTqDemFr_Nm] -> Add5/1
  Add5/1 -> Relational Operator10/1
  Constant26/1 -> Switch10/3
  Constant25/1 -> Relational Operator10/2
  Switch1/1 -> Product/2
  Switch10/1 -> Product/1

== system vmc/VMC/VMC/SpeedArbitration/Feature Arbitration ==
  VVMC_FeatStaConfirm_enum : Inport
  VDSC_DISCTargetSpd_kph : Inport  Port=2
  VVMC_FeatSetSpdForCalcu_kph : Inport  Port=3
  VVMC_LastFeatArbitrFinal_enum : Inport  Port=4
  VVMC_LastActACCRequiredAccel_mps2 : Inport  Port=5
  Constant1 : Constant  Value=ENUM_FEATSTACFM_AEB
  Constant10 : Constant  Value=ENUM_FEATARBITRSTA_AEB
  Constant11 : Constant  Value=ENUM_FEATARBITRSTA_ACC
  Constant12 : Constant  Value=ENUM_FEATARBITRSTA_CC
  Constant13 : Constant  Value=ENUM_FEATARBITRSTA_DISC
  Constant14 : Constant  Value=ENUM_FEATARBITRSTA_MSA
  Constant15 : Constant  Value=ZERO_FLOAT
  Constant18 : Constant  Value=ENUM_FEATARBITRSTA_ACCDISC
  Constant2 : Constant  Value=ENUM_FEATSTACFM_ACC
  Constant3 : Constant  Value=ENUM_FEATSTACFM_CC
  Constant4 : Constant  Value=ENUM_FEATSTACFM_DISC
  Constant5 : Constant  Value=ENUM_FEATSTACFM_MSA
  Constant6 : Constant  Value=ENUM_FEATSTACFM_ACCDISC
  Constant7 : Constant  Value=ENUM_FEATSTACFM_CCDISC
  Constant8 : Constant  Value=ENUM_FEATSTACFM_DISCMSA
  Constant9 : Constant  Value=ENUM_FEATARBITRSTA_INACTIVE
  Feature Arbitration : Stateflow chart  TreatAsAtomicUnit=on
      settings: PortSchema="{\"entries\":[{\"content\":{\"sides\":[{\"content\":{\"connectorIds\":[\"In1\",\"In2\",\"In3\",\"In4\",\"In5\",\"In6\",\"In7\",\"In8\",\"In9\",\"In10\",\"In11\",\"In12\",\"In13\",\"In14\",\"In15\",\"In16\",\"In17\",\"In18\",\"In19\",\"In21\",\"In20\"]},\"type\":\"ConnectorPlacement.EquallySpacedRectSide\",\"uuid\":\"aab57011-fcd5-4ecf-9d9a-0c506a56b983\"},{\"content\":{\"connectorIds\":[\"Out1\",\"Out2\"],\"side\":\"RIGHT\"},\"type\":\"ConnectorPlacement.EquallySpacedRectSide\",\"uuid\":\"91772277-5a1b-49e4-a418-6bbcd6aa0e8d\"},{\"content\":{\"connectorIds\":[],\"side\":\"TOP\"},\"type\":\"ConnectorPlacement.EquallySpacedRectSide\",\"uuid\":\"5425f30d-bcbe-40de-8bf0-3b50206f90f2\"}]},\"type\":\"ConnectorPlacement.EquallySpacedConnector\",\"uuid\":\"f1fd0360-59b6-41b6-975b-0f3df9568038\"}],\"packageUris\":[\"http://schema.mathworks.com/mf0/Connector/R2020b\"],\"version\":\"1.0\"}"
  VVMC_FeatArbitrSta_enum : Outport
  VVMC_FeatReqSpd_kph : Outport  Port=2
  wires:
  Constant18/1 -> Feature Arbitration/17(ENUM_FEATARBITRSTA_ACCDISC)
  Constant15/1 -> Feature Arbitration/19(ZERO_FLOAT)
  Constant14/1 -> Feature Arbitration/18(ENUM_FEATARBITRSTA_MSA)
  Constant13/1 -> Feature Arbitration/16(ENUM_FEATARBITRSTA_DISC)
  Constant12/1 -> Feature Arbitration/15(ENUM_FEATARBITRSTA_CC)
  Constant11/1 -> Feature Arbitration/14(ENUM_FEATARBITRSTA_ACC)
  Constant10/1 -> Feature Arbitration/13(ENUM_FEATARBITRSTA_AEB)
  Constant9/1 -> Feature Arbitration/12(ENUM_FEATARBITRSTA_INACTIVE)
  Constant8/1 -> Feature Arbitration/11(ENUM_FEATSTACFM_DISCMSA)
  Constant7/1 -> Feature Arbitration/10(ENUM_FEATSTACFM_CCDISC)
  Constant6/1 -> Feature Arbitration/9(ENUM_FEATSTACFM_ACCDISC)
  Constant5/1 -> Feature Arbitration/8(ENUM_FEATSTACFM_MSA)
  Constant4/1 -> Feature Arbitration/7(ENUM_FEATSTACFM_DISC)
  Constant3/1 -> Feature Arbitration/6(ENUM_FEATSTACFM_CC)
  Constant2/1 -> Feature Arbitration/5(ENUM_FEATSTACFM_ACC)
  Constant1/1 -> Feature Arbitration/4(ENUM_FEATSTACFM_AEB)
  [VVMC_FeatReqSpd_kph] -> VVMC_FeatReqSpd_kph/1
  [VVMC_FeatArbitrSta_enum] -> VVMC_FeatArbitrSta_enum/1
  Feature Arbitration/2(VVMC_FeatReqSpd_kph) -> [VVMC_FeatReqSpd_kph]
  Feature Arbitration/1(VVMC_FeatArbitrSta_enum) -> [VVMC_FeatArbitrSta_enum]
  [VVMC_FeatSetSpdForCalcu_kph] -> Feature Arbitration/3(VVMC_FeatSetSpdForCalcu_kph)
  [VDSC_DISCTargetSpd_kph] -> Feature Arbitration/2(VDSC_DISCTargetSpd_kph)
  [VVMC_FeatStaConfirm_enum] -> Feature Arbitration/1(VVMC_FeatStaConfirm_enum)
  VVMC_FeatSetSpdForCalcu_kph/1 -> [VVMC_FeatSetSpdForCalcu_kph]
  VDSC_DISCTargetSpd_kph/1 -> [VDSC_DISCTargetSpd_kph]
  VVMC_FeatStaConfirm_enum/1 -> [VVMC_FeatStaConfirm_enum]
  VVMC_LastFeatArbitrFinal_enum/1 -> [VVMC_LastFeatArbitrFinal_enum]
  VVMC_LastActACCRequiredAccel_mps2/1 -> [VVMC_LastActACCRequiredAccel_mps2]
  [VVMC_LastActACCRequiredAccel_mps2] -> Feature Arbitration/20(VVMC_LastActACCRequiredAccel_mps2)
  [VVMC_LastFeatArbitrFinal_enum] -> Feature Arbitration/21(VVMC_LastFeatArbitrFinal_enum)

== system vmc/VMC/VMC/SpeedArbitration/Feature Status Confirm ==
  VVMC_VMCCCCtrlAvail_flg : Inport
  VVMC_VMCMSACtrlAvail_flg : Inport  Port=2
  VVMC_VMCAEBCtrlAvail_flg : Inport  Port=3
  VVMC_VMCACCCtrlAvail_flg : Inport  Port=4
  VINP_ADASAEBSta_enum : Inport  Port=5
  VDSC_DISCSta_enum : Inport  Port=6
  VINP_ADASACCSta_enum : Inport  Port=7
  VVMC_CCCtrlSta_enum : Inport  Port=8
  VVMC_MSACtrlSta_enum : Inport  Port=9
  VINP_ADASAEBReq_enum : Inport  Port=10
  Constant : Constant  Value=ENUM_FEATSTACFM_INACTIVE
  Constant1 : Constant  Value=ENUM_FEATSTACFM_AEB
  Constant10 : Constant  Value=ENUM_VMCAEBCTRLAVAIL_AVAILABLE
  Constant11 : Constant  Value=ENUM_CCCRLSTA_ACTIVE
  Constant12 : Constant  Value=ENUM_ADASMSASTA_ACTIVE
  Constant13 : Constant  Value=ENUM_DISCSTA_ACTIVE
  Constant14 : Constant  Value=ENUM_ADASAEBSTA_ACTIVE
  Constant15 : Constant  Value=ENUM_VMCACCCTRLAVAIL_AVAILABLE
  Constant16 : Constant  Value=ENUM_VMCMSACTRLAVAIL_AVAILABLE
  Constant17 : Constant  Value=ENUM_VMCCCCTRLAVAIL_AVAILABLE
  Constant18 : Constant  Value=ENUM_ADASACCSTA_SHUTOFF
  Constant19 : Constant  Value=ENUM_ADASACCSTA_OVERRIDE
  Constant2 : Constant  Value=ENUM_FEATSTACFM_ACC
  Constant20 : Constant  Value=ENUM_ADASAEBREQ_NOREQUEST
  Constant21 : Constant  Value=ENUM_CCCRLSTA_OVERRIDE
  Constant22 : Constant  Value=ENUM_ADASMSASTA_UNLIMIT
  Constant3 : Constant  Value=ENUM_FEATSTACFM_CC
  Constant4 : Constant  Value=ENUM_FEATSTACFM_DISC
  Constant5 : Constant  Value=ENUM_FEATSTACFM_MSA
  Constant6 : Constant  Value=ENUM_FEATSTACFM_ACCDISC
  Constant7 : Constant  Value=ENUM_FEATSTACFM_CCDISC
  Constant8 : Constant  Value=ENUM_FEATSTACFM_DISCMSA
  Constant9 : Constant  Value=ENUM_ADASACCSTA_ACTIVE
  Feature Status Confirm : Stateflow chart  TreatAsAtomicUnit=on
  VVMC_FeatStaConfirm_enum : Outport
  wires:
  Constant20/1 -> Feature Status Confirm/31(ENUM_ADASAEBREQ_NOREQUEST)
  [VINP_ADASAEBReq_enum] -> Feature Status Confirm/30(VINP_ADASAEBReq_enum)
  VINP_ADASAEBReq_enum/1 -> [VINP_ADASAEBReq_enum]
  Constant19/1 -> Feature Status Confirm/29(ENUM_ADASACCSTA_OVERRIDE)
  Constant18/1 -> Feature Status Confirm/25(ENUM_ADASACCSTA_SHUTOFF)
  [VVMC_VMCCCCtrlAvail_flg] -> Feature Status Confirm/1(VVMC_VMCCCCtrlAvail_flg)
  Constant17/1 -> Feature Status Confirm/2(ENUM_VMCCCCTRLAVAIL_AVAILABLE)
  [VVMC_VMCMSACtrlAvail_flg] -> Feature Status Confirm/3(VVMC_VMCMSACtrlAvail_flg)
  Constant16/1 -> Feature Status Confirm/4(ENUM_VMCMSACTRLAVAIL_AVAILABLE)
  VVMC_VMCMSACtrlAvail_flg/1 -> [VVMC_VMCMSACtrlAvail_flg]
  VVMC_VMCCCCtrlAvail_flg/1 -> [VVMC_VMCCCCtrlAvail_flg]
  [VVMC_VMCAEBCtrlAvail_flg] -> Feature Status Confirm/5(VVMC_VMCAEBCtrlAvail_flg)
  Constant10/1 -> Feature Status Confirm/6(ENUM_VMCAEBCTRLAVAIL_AVAILABLE)
  [VVMC_VMCACCCtrlAvail_flg] -> Feature Status Confirm/7(VVMC_VMCACCCtrlAvail_flg)
  Constant15/1 -> Feature Status Confirm/8(ENUM_VMCACCCTRLAVAIL_AVAILABLE)
  VVMC_VMCAEBCtrlAvail_flg/1 -> [VVMC_VMCAEBCtrlAvail_flg]
  VVMC_VMCACCCtrlAvail_flg/1 -> [VVMC_VMCACCCtrlAvail_flg]
  Constant14/1 -> Feature Status Confirm/23(ENUM_ADASAEBSTA_ACTIVE)
  Constant13/1 -> Feature Status Confirm/28(ENUM_DISCSTA_ACTIVE)
  Constant12/1 -> Feature Status Confirm/27(ENUM_MSACRLSTA_ACTIVE)
  Constant11/1 -> Feature Status Confirm/26(ENUM_CCCRLSTA_ACTIVE)
  Constant9/1 -> Feature Status Confirm/24(ENUM_ADASACCSTA_ACTIVE)
  Constant8/1 -> Feature Status Confirm/22(ENUM_FEATSTACFM_DISCMSA)
  Constant7/1 -> Feature Status Confirm/21(ENUM_FEATSTACFM_CCDISC)
  Constant6/1 -> Feature Status Confirm/20(ENUM_FEATSTACFM_ACCDISC)
  Constant5/1 -> Feature Status Confirm/19(ENUM_FEATSTACFM_MSA)
  Constant4/1 -> Feature Status Confirm/18(ENUM_FEATSTACFM_DISC)
  Constant3/1 -> Feature Status Confirm/17(ENUM_FEATSTACFM_CC)
  Constant2/1 -> Feature Status Confirm/16(ENUM_FEATSTACFM_ACC)
  Constant1/1 -> Feature Status Confirm/15(ENUM_FEATSTACFM_AEB)
  Constant/1 -> Feature Status Confirm/14(ENUM_FEATSTACFM_INACTIVE)
  [VVMC_FeatStaConfirm_enum] -> VVMC_FeatStaConfirm_enum/1
  Feature Status Confirm/1(VVMC_FeatStaConfirm_enum) -> [VVMC_FeatStaConfirm_enum]
  VVMC_MSACtrlSta_enum/1 -> [VVMC_MSACtrlSta_enum]
  VVMC_CCCtrlSta_enum/1 -> [VVMC_CCCtrlSta_enum]
  VINP_ADASACCSta_enum/1 -> [VINP_ADASACCSta_enum]
  VDSC_DISCSta_enum/1 -> [VDSC_DISCSta_enum]
  VINP_ADASAEBSta_enum/1 -> [VINP_ADASAEBSta_enum]
  [VVMC_CCCtrlSta_enum] -> Feature Status Confirm/12(VVMC_CCCtrlSta_enum)
  [VINP_ADASAEBSta_enum] -> Feature Status Confirm/9(VINP_ADASAEBSta_enum)
  [VINP_ADASACCSta_enum] -> Feature Status Confirm/11(VINP_ADASACCSta_enum)
  [VDSC_DISCSta_enum] -> Feature Status Confirm/10(VDSC_DISCSta_enum)
  [VVMC_MSACtrlSta_enum] -> Feature Status Confirm/13(VVMC_MSACtrlSta_enum)
  Constant22/1 -> Feature Status Confirm/33(ENUM_MSACRLSTA_OVERRIDE)
  Constant21/1 -> Feature Status Confirm/32(ENUM_CCCRLSTA_OVERRIDE)

== system vmc/VMC/VMC/SpeedArbitration/Response Gain ==
  VDSC_DISCTurn_flg : Inport
  VVMC_FeatArbitrSta_enum : Inport  Port=2
  VVMC_FeatReqSpd_kph : Inport  Port=3
  VVMC_MeterIndSpeedForCalcu_kph : Inport  Port=4
  VINP_VehSpeed_kph : Inport  Port=5
  VDSC_AutoTurnMode_flg : Inport  Port=6
  VDSC_DISCTargetSpd_kph : Inport  Port=7
  Abs : Abs
  Add : Sum  Inputs=-+
  Add4 : Sum
  Constant1 : Constant  Value=KVMC_Veh2MeterSpdFactor_enum
  Constant13 : Constant  Value=ENUM_FEATARBITRSTA_DISC
  Constant15 : Constant  Value=ZERO_FLOAT
  Constant16 : Constant  Value=ENUM_DISCTURN_ACTIVE
  Constant18 : Constant  Value=ENUM_FEATARBITRSTA_ACCDISC
  Constant2 : Constant  Value=ENUM_FEATARBITRSTA_CC
  Constant23 : Constant  Value=KVMC_Veh2MeterSpdOffset_enum
  Constant28 : Constant  Value=KVMC_Veh2MeterSpdLoFactor_enum
  Constant3 : Constant  Value=ENUM_FEATARBITRSTA_MSA
  Constant4 : Constant  Value=TRUE
  Constant5 : Constant  Value=KVMC_MSAResponseAGSV_flg
  Divide5 : Product  Inputs=**
  Divide8 : Product  Inputs=**
  MVMC_AggressJerkPCT4AT_pct : Lookup_n-D  NumberOfTableDimensions=1  BreakpointsForDimension1=AVMC_AggressJerkPCT4AT_X_kph  Table=MVMC_AggressJerkPCT4AT_Y_pct  InternalRulePriority=Speed  RndMeth=Simplest  InputSameDT=on
  MVMC_AggressJerkPCT_pct : Lookup_n-D  NumberOfTableDimensions=1  BreakpointsForDimension1=AVMC_AggressJerkPCT_X_kph  Table=MVMC_AggressJerkPCT_Y_pct  InternalRulePriority=Speed  RndMeth=Simplest  InputSameDT=on
  MVMC_AggressJerkPCT_pct1 : Lookup_n-D  NumberOfTableDimensions=1  BreakpointsForDimension1=AVMC_AggressJerkPCT_X_kph  Table=MVMC_AggressJerkPCT_Y_pct  InternalRulePriority=Speed  RndMeth=Simplest  InputSameDT=on
  MVMC_AggressLimitPCT4AT_pct : Lookup_n-D  NumberOfTableDimensions=1  BreakpointsForDimension1=AVMC_AggressLimitPCT4AT_X_kph  Table=MVMC_AggressLimitPCT4AT_Y_pct  InternalRulePriority=Speed  RndMeth=Simplest  InputSameDT=on
  MVMC_AggressLimitPCT_pct : Lookup_n-D  NumberOfTableDimensions=1  BreakpointsForDimension1=AVMC_AggressLimitPCT_X_kph  Table=MVMC_AggressLimitPCT_Y_pct  InternalRulePriority=Speed  RndMeth=Simplest  InputSameDT=on
  MVMC_AggressLimitPCT_pct1 : Lookup_n-D  NumberOfTableDimensions=1  BreakpointsForDimension1=AVMC_AggressLimitPCT_X_kph  Table=MVMC_AggressLimitPCT_Y_pct  InternalRulePriority=Speed  RndMeth=Simplest  InputSameDT=on
  MVMC_SoftJerkPCT_pct : Lookup_n-D  NumberOfTableDimensions=1  BreakpointsForDimension1=AVMC_SoftJerkPCT_X_kph  Table=MVMC_SoftJerkPCT_Y_pct  InternalRulePriority=Speed  RndMeth=Simplest  InputSameDT=on
  MVMC_SoftLimitPCT_pct : Lookup_n-D  NumberOfTableDimensions=1  BreakpointsForDimension1=AVMC_SoftLimitPCT_X_kph  Table=MVMC_SoftLimitPCT_Y_pct  InternalRulePriority=Speed  RndMeth=Simplest  InputSameDT=on
  Relational Operator : RelationalOperator  Operator=>  OutDataTypeStr=boolean  RndMeth=Simplest
  Relational Operator1 : RelationalOperator  Operator=>  OutDataTypeStr=boolean  RndMeth=Simplest
  Response Gain : Stateflow chart  TreatAsAtomicUnit=on
  Switch : Switch  Criteria=u2 > Threshold  Threshold=KVMC_Veh2MeterSpdLoBdy_kph
  Switch{1..4} (4 alike) : Switch  Criteria=u2 > Threshold
  VVMC_JerkPCT_pct : Outport
  VVMC_LimitPCT_pct : Outport  Port=2
  wires:
  Switch/1 -> Add/1
  VINP_VehSpeed_kph/1 -> [VINP_VehSpeed_kph]
  Abs/1 -> MVMC_SoftLimitPCT_pct/1, MVMC_AggressLimitPCT_pct1/1, MVMC_AggressLimitPCT4AT_pct/1, MVMC_AggressLimitPCT_pct/1
  Add/1 -> Abs/1
  [VVMC_FeatReqSpd_kph] -> Add/2
  VVMC_FeatReqSpd_kph/1 -> [VVMC_FeatReqSpd_kph]
  Switch1/1 -> [VVMC_AggressLimitPCT_pct]  "VVMC_AggressLimitPCT_pct"
  MVMC_SoftLimitPCT_pct/1 -> [VVMC_SoftLimitPCT_pct]  "VVMC_SoftLimitPCT_pct"
  Switch2/1 -> [VVMC_AggressJerkPCT_pct]  "VVMC_AggressJerkPCT_pct"
  MVMC_SoftJerkPCT_pct/1 -> [VVMC_SoftJerkPCT_pct]  "VVMC_SoftJerkPCT_pct"
  [VVMC_MeterIndSpeedForCalcu_kph] -> MVMC_SoftJerkPCT_pct/1, MVMC_AggressJerkPCT4AT_pct/1, MVMC_AggressJerkPCT_pct/1, MVMC_AggressJerkPCT_pct1/1
  VVMC_MeterIndSpeedForCalcu_kph/1 -> [VVMC_MeterIndSpeedForCalcu_kph]
  Constant18/1 -> Response Gain/11(ENUM_FEATARBITRSTA_ACCDISC)
  Constant16/1 -> Response Gain/10(ENUM_DISCTURN_ACTIVE)
  Constant15/1 -> Response Gain/9(ZERO_FLOAT)
  Constant13/1 -> Response Gain/7(ENUM_FEATARBITRSTA_DISC)
  [VVMC_LimitPCT_pct] -> VVMC_LimitPCT_pct/1
  [VVMC_JerkPCT_pct] -> VVMC_JerkPCT_pct/1
  [VVMC_AggressLimitPCT_pct] -> Response Gain/6(VVMC_AggressLimitPCT_pct)
  [VVMC_SoftLimitPCT_pct] -> Response Gain/5(VVMC_SoftLimitPCT_pct)
  [VVMC_AggressJerkPCT_pct] -> Response Gain/4(VVMC_AggressJerkPCT_pct)
  [VVMC_SoftJerkPCT_pct] -> Response Gain/3(VVMC_SoftJerkPCT_pct)
  [VVMC_FeatArbitrSta_enum] -> Response Gain/2(VVMC_FeatArbitrSta_enum)
  VVMC_FeatArbitrSta_enum/1 -> [VVMC_FeatArbitrSta_enum]
  VDSC_DISCTurn_flg/1 -> [VDSC_DISCTurn_flg]
  Response Gain/2(VVMC_LimitPCT_pct) -> [VVMC_LimitPCT_pct]
  [VDSC_DISCTurn_flg] -> Response Gain/1(VDSC_DISCTurn_flg)
  Response Gain/1(VVMC_JerkPCT_pct) -> [VVMC_JerkPCT_pct]
  Constant23/1 -> Add4/1
  Divide8/1 -> Switch/3
  Constant28/1 -> Divide8/2
  Add4/1 -> Switch/1
  Divide5/1 -> Add4/2
  [VINP_VehSpeed_kph] -> Switch/2, Divide8/1, Divide5/2
  Constant1/1 -> Divide5/1
  Constant2/1 -> Response Gain/8(ENUM_FEATARBITRSTA_CC)
  Constant3/1 -> Response Gain/12(ENUM_FEATARBITRSTA_MSA)
  Constant4/1 -> Response Gain/13(TRUE)
  Constant5/1 -> Response Gain/14(KVMC_MSAResponseAGSV_flg)
  VDSC_AutoTurnMode_flg/1 -> [VDSC_AutoTurnMode_flg]
  [VDSC_AutoTurnMode_flg] -> Switch2/2
  MVMC_AggressJerkPCT_pct/1 -> Switch2/3
  MVMC_AggressJerkPCT4AT_pct/1 -> Switch4/3
  [VDSC_AutoTurnMode_flg] -> Switch1/2
  MVMC_AggressLimitPCT_pct/1 -> Switch1/3
  MVMC_AggressLimitPCT4AT_pct/1 -> Switch3/3
  VDSC_DISCTargetSpd_kph/1 -> [VDSC_DISCTargetSpd_kph]
  [VVMC_MeterIndSpeedForCalcu_kph] -> Relational Operator/2
  [VDSC_DISCTargetSpd_kph] -> Relational Operator/1
  Relational Operator/1 -> Switch3/2
  MVMC_AggressLimitPCT_pct1/1 -> Switch3/1
  Switch3/1 -> Switch1/1
  Switch4/1 -> Switch2/1
  MVMC_AggressJerkPCT_pct1/1 -> Switch4/1
  Relational Operator1/1 -> Switch4/2
  [VDSC_DISCTargetSpd_kph] -> Relational Operator1/1
  [VVMC_MeterIndSpeedForCalcu_kph] -> Relational Operator1/2
